simulink model "DEC_LA2"  (R2015a)
settings: Solver=ode5  StartTime=0  StopTime=sim_time-1/sr  FixedStep=1/sr  RelTol=1e-3
values from neighbouring files (symbols this model uses):
  par = p.Results.par_fix    [balance_sim.m]
settings Model: Creator=lorenz  LastModifiedBy=lorenz
settings DataIOCC: LimitDataPoints=off  SignalLoggingSaveFormat=ModelDataLogs  SaveOutput=off  SignalLogging=off  DSMLogging=off  SaveTime=off
settings OptimizationCC: OptimizeBlockIOStorage=off  BufferReuse=off  GlobalBufferReuse=off  ExpressionFolding=off  LocalBlockOutputs=off
settings DebuggingCC: UnderspecifiedInitializationDetection=Classic  SolverPrmCheckMsg=warning  InheritedTsInSrcMsg=none  MultiTaskDSMMsg=warning  MultiTaskCondExecSysMsg=none
settings ModelReferenceCC: UpdateModelReferenceTargets=AssumeUpToDate  CheckModelReferenceTargetMessage=warning
settings RTWCC: ProfileTLC=on  RTWUseSimCustomCode=on
settings CodeAppCC: MATLABSourceComments=on

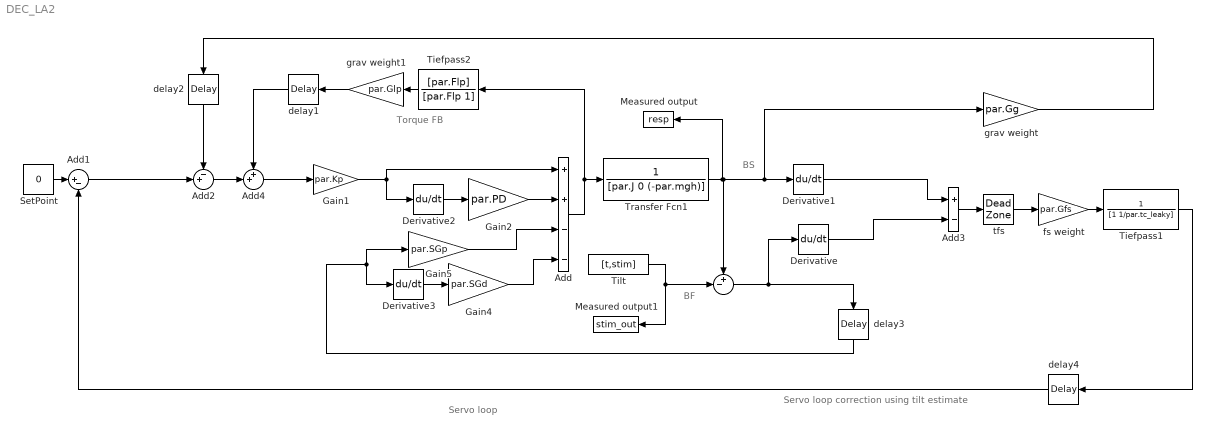
== system DEC_LA2 ==
  note: Servo loop
  note: BS
  note: BF
  note: Torque FB
  note: Servo loop correction using tilt estimate
  " " : Sum  Inputs=+-|
  Add : Sum  Inputs=++--
  Add1 : Sum  Inputs=|+-
  Add2 : Sum  Inputs=-+|
  Add3 : Sum  Inputs=+-
  Add4 : Sum  Inputs=++|
  Derivative{,1..3} (4 alike) : Derivative
  Gain1 : Gain  Gain=par.Kp
  Gain2 : Gain  Gain=par.PD
  Gain4 : Gain  Gain=par.SGd
  Gain5 : Gain  Gain=par.SGp
  Measured output : ToWorkspace  VariableName=resp  SampleTime=-1
  Measured output1 : ToWorkspace  VariableName=stim_out  SampleTime=-1
  SetPoint : Constant  Value=0
  Tiefpass1 : TransferFcn  Denominator=[1 1/par.tc_leaky]
  Tiefpass2 : TransferFcn  Numerator=[par.Flp]  Denominator=[par.Flp 1]
  Tilt : FromWorkspace  VariableName=[t,stim]
  Transfer Fcn1 : TransferFcn  Denominator=[par.J 0 (-par.mgh)]
  delay1 : TransportDelay  DelayTime=par.dt  FixedBuffer=on
  delay2 : TransportDelay  DelayTime=par.dt  FixedBuffer=on
  delay3 : TransportDelay  DelayTime=par.dt2  FixedBuffer=on
  delay4 : TransportDelay  DelayTime=par.dt  FixedBuffer=on
  fs weight : Gain  Gain=par.Gfs
  grav weight : Gain  Gain=par.Gg
  grav weight1 : Gain  Gain=par.Glp
  tfs : DeadZone  LowerValue=-par.tfs  UpperValue=par.tfs  LinearizeAsGain=off
  wires:
  delay4/1 -> Add1/2
  SetPoint/1 -> Add1/1
  tfs/1 -> fs weight/1
  fs weight/1 -> Tiefpass1/1
  Derivative1/1 -> Add3/1
  Derivative/1 -> Add3/2
  Add3/1 -> tfs/1
  Tiefpass1/1 -> delay4/1
  grav weight/1 -> delay2/1
  Tiefpass2/1 -> grav weight1/1
  " "/1 -> delay3/1, Derivative/1
  Add2/1 -> Add4/2
  Transfer Fcn1/1 -> Derivative1/1, grav weight/1, " "/1, Measured output/1
  Add/1 -> Tiefpass2/1, Transfer Fcn1/1
  Tilt/1 -> " "/2, Measured output1/1
  grav weight1/1 -> delay1/1
  Add4/1 -> Gain1/1
  Derivative2/1 -> Gain2/1
  Gain2/1 -> Add/2
  Gain1/1 -> Derivative2/1, Add/1
  delay1/1 -> Add4/1
  delay2/1 -> Add2/1
  Add1/1 -> Add2/2
  Derivative3/1 -> Gain4/1
  delay3/1 -> Gain5/1, Derivative3/1
  Gain4/1 -> Add/4
  Gain5/1 -> Add/3
